simulink model "Model_LQI"  (R2025b)
settings: Solver=VariableStepAuto  StartTime=0.0  StopTime=10.0  RelTol=1e-3
PreLoadFcn:
  | setup_sim_LQI
InitFcn:
  | setup_sim_LQI
values from neighbouring files (symbols this model uses):
  hover_throttle = round(exact_throttle)    [setup_sim.m]    (also in setup_sim_LQI.m = round(exact_throttle) / 10; setup_sim_PID.m)
undefined symbols (not defined in the file or in its folder): config, DiscIntNeverNeededParam, params
settings Model: Creator=samue  LastModifiedBy=samue

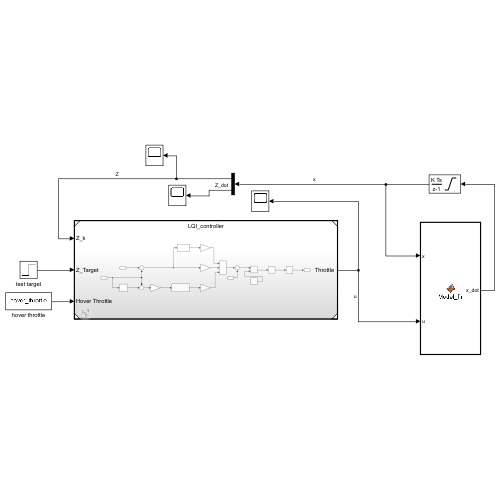
[thumbnail: Simulink's stored preview of the top-level diagram]
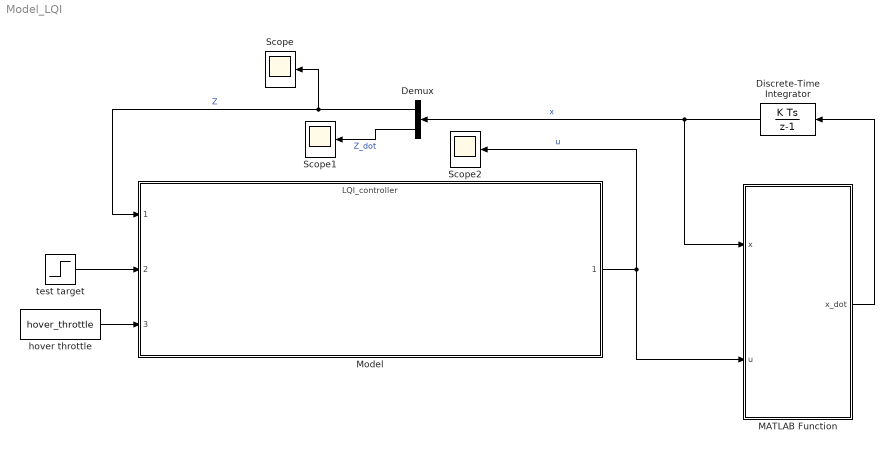
== system Model_LQI ==
  Demux : Demux  Outputs=2
  Discrete-Time Integrator : DiscreteIntegrator  InitialCondition=[config.initial_height;0]  SampleTime=-1  LimitOutput=on  UpperSaturationLimit=params.max_height  LowerSaturationLimit=params.min_height  ICPrevOutput=DiscIntNeverNeededParam  ICPrevScaledInput=DiscIntNeverNeededParam
  MATLAB Function : MATLAB Function  TreatAsAtomicUnit=on
  Model : ModelReference  ModelNameDialog=LQI_controller.slx  SimulationMode=Normal  ModelReferenceVersion=1.19
  Scope : Scope
      settings: ActiveDisplayYMinimum=0.029592869109643871  ActiveDisplayYMaximum=1.8978153778952063
  Scope1 : Scope
      settings: ActiveDisplayYMinimum=0.029592869109643871  ActiveDisplayYMaximum=1.8978153778952063
  Scope2 : Scope
      settings: ActiveDisplayYMinimum=-50.289073562933993  ActiveDisplayYMaximum=272.26171493064771  DataLoggingVariableName=ScopeData2
  hover throttle : Constant  Value=hover_throttle
  test target : Step  Time=0  SampleTime=0
  wires:
  test target/1 -> Model/2
  Discrete-Time Integrator/1 -> MATLAB Function/1(x), Demux/1  "x"
  Model/1 -> Scope2/1, MATLAB Function/2(u)  "u"
  MATLAB Function/1(x_dot) -> Discrete-Time Integrator/1
  hover throttle/1 -> Model/3
  Demux/1 -> Scope/1, Model/1  "Z"
  Demux/2 -> Scope1/1  "Z_dot"

== matlab function Model_LQI/MATLAB Function ==
  data: x input; u input; x_dot output; config parameter; params parameter
function x_dot = Model_fn(x, u, config, params)
    x_dot = physics_model(x, u, config, params);
end
